simulink model "DC_Motor"  (R2020b)
settings: Solver=VariableStepAuto  StartTime=0.0  StopTime=10.0  RelTol=1e-3
undefined symbols (not defined in the file or in its folder): b, J, K, L, R
settings Model: Creator=shoun  LastModifiedBy=shoun

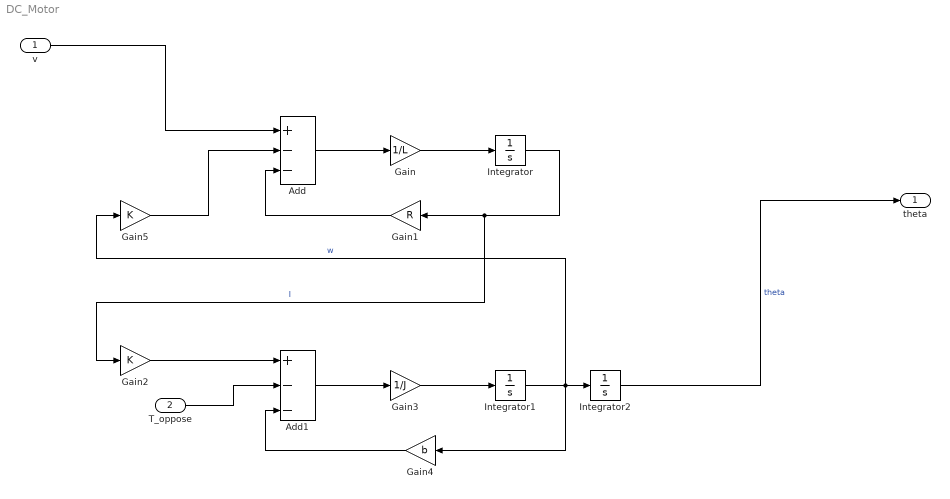
== system DC_Motor ==
  v : Inport  OutDataTypeStr=double  PortDimensions=1  SampleTime=0
  T_oppose : Inport  Port=2  OutDataTypeStr=double  PortDimensions=1
  Add : Sum  Inputs=+--
  Add1 : Sum  Inputs=+--
  Gain : Gain  Gain=1/L
  Gain1 : Gain  Gain=R
  Gain2 : Gain  Gain=K
  Gain3 : Gain  Gain=1/J
  Gain4 : Gain  Gain=b
  Gain5 : Gain  Gain=K
  Integrator : Integrator
  Integrator1 : Integrator
  Integrator2 : Integrator
  theta : Outport  OutDataTypeStr=double  PortDimensions=1  SampleTime=0
  wires:
  Integrator1/1 -> Integrator2/1, Gain5/1, Gain4/1  "w"
  Gain5/1 -> Add/2
  T_oppose/1 -> Add1/2
  Integrator2/1 -> theta/1  "theta"
  Gain4/1 -> Add1/3
  Gain/1 -> Integrator/1
  Integrator/1 -> Gain1/1, Gain2/1  "I"
  Gain1/1 -> Add/3
  Gain2/1 -> Add1/1
  v/1 -> Add/1
  Add1/1 -> Gain3/1
  Add/1 -> Gain/1
  Gain3/1 -> Integrator1/1
